simulink model "nomal_regulator"  (R2019a)
settings: Solver=FixedStepAuto  StartTime=0.0  StopTime=20  FixedStep=sT  RelTol=1e-3
InitFcn:
  | param;
values from neighbouring files (symbols this model uses):
  A = [0 1; w^2 0]    [continus.m]    (also in discrete.m = [0 1; omega^2 0]; param.m = [0 1; omega^2 0]; param2.m = [0 1; omega^2 0]; param_kf.m)
  B = [0; -w^2]    [continus.m]    (also in discrete.m = [0; -omega^2]; param.m = [0; -omega^2]; param2.m = [0; -omega^2]; param_kf.m)
  C = eye(2)    [discrete.m]    (also in param.m; param2.m; param_kf.m = [w^2 0]; test0.m)
  D = [0 0]'    [discrete.m]    (also in param.m; param2.m; param_kf.m = -w^2; test0.m)
  inix = [0.00 0.0]'    [param.m]    (also in param2.m = [0.05 0.0]'; param_kf.m = [0.0 0.0]')
  K = [k1 k2]    [continus.m]    (also in discrete.m = -place(A, B, [q1 q2]); param.m; param2.m = dlqr(A,B,Q,H); param_kf.m = -place(A, B, [q1 q2]))
settings Model: Creator=hideaki  LastModifiedBy=hideaki

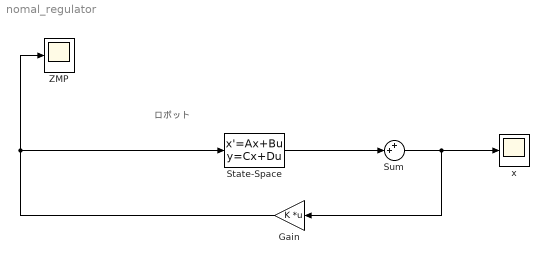
== system nomal_regulator ==
  note: ロボット
  Gain : Gain  Gain=K  Multiplication=Matrix(K*u)
  State-Space : StateSpace  A=A  B=B  C=C  D=D  InitialCondition=inix
  Sum : Sum  Inputs=++|
  ZMP : Scope
  x : Scope
  wires:
  Sum/1 -> x/1, Gain/1
  Gain/1 -> ZMP/1, State-Space/1
  State-Space/1 -> Sum/2
